simulink model "practica2"  (R2014a)
settings: Solver=ode45  StartTime=0.0  StopTime=10.0  RelTol=1e-3
undefined symbols (not defined in the file): get
libraries: dsparch4 x2, dspsrcs4 x2, dspspect3 x1, dspsnks4 x1
settings Model: Creator=MANU  LastModifiedBy=Isabela

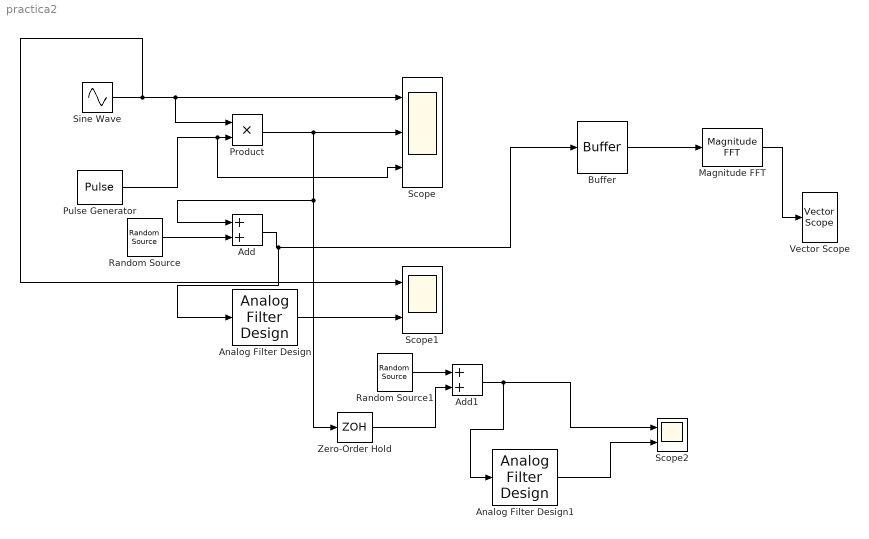
== system practica2 ==
  Add : Sum
  Add1 : Sum
  Analog Filter Design : dsparch4/Analog Filter Design  method=Butterworth  filttype=Lowpass  N=80  Wlo=30  Whi=80  Rp=2  Rs=40
  Analog Filter Design1 : dsparch4/Analog Filter Design  method=Butterworth  filttype=Lowpass  N=30  Wlo=200  Whi=80  Rp=2  Rs=40
  Buffer : Buffer  TreatMby1Signals=One channel
  Magnitude FFT : dspspect3/Magnitude FFT  mag_or_magsq=Magnitude squared  FFTImplementation=Auto  fftLenInherit=off  fftsize=256  WrapInput=on
  Product : Product  RndMeth=Zero
  Pulse Generator : DiscretePulseGenerator  Amplitude=2  Period=3  SampleTime=0.01
  Random Source : dspsrcs4/Random Source  SrcType=Gaussian  NormMethod=Sum of uniform values  CltLength=4  MinVal=0  MaxVal=2  MeanVal=0  VarVal=0.5  RepMode=Not repeatable  rawSeed=1  IsInherit=off  SampMode=Discrete  SampTime=1  SampFrame=1  DataType=Double  OutComplex=Real
  Random Source1 : dspsrcs4/Random Source  SrcType=Gaussian  NormMethod=Sum of uniform values  CltLength=4  MinVal=0  MaxVal=2  MeanVal=0  VarVal=0.5  RepMode=Not repeatable  rawSeed=1  IsInherit=off  SampMode=Discrete  SampTime=1  SampFrame=1  DataType=Double  OutComplex=Real
  Scope : Scope  NumInputPorts=3
      settings: YMin=-5~-5~-5  YMax=5~5~5
  Scope1 : Scope  NumInputPorts=2
      settings: YMin=-5~-5  YMax=5~5
  Scope2 : Scope  NumInputPorts=2
      settings: YMin=-5~-5  YMax=5~5  SaveName=ScopeData2
  Sine Wave : Sin  SineType=Sample based  Amplitude=10  Frequency=5  Samples=60  SampleTime=0.01
  Vector Scope : dspsnks4/Vector Scope  ScopeProperties=on  Domain=Time  HorizSpan=1  DisplayProperties=off  AxisGrid=on  Memory=off  FrameNumber=on  AxisLegend=off  AxisZoom=off  OpenScopeAtSimStart=on  OpenScopeImmediately=off  FigPos=get(0,'defaultfigureposition')  AxisProperties=off  XUnits=Hertz  XRange=[0...Fs/2]  InheritXIncr=on  XIncr=1  XLabel=Time  XLimit=Auto  XMin=0  XMax=1  XStart=0  YUnits=dB  YLabel=Amplitude  LineProperties=off  XAxisParamsVer=6.9
      settings: YMin=-10  YMax=10
  Zero-Order Hold : ZeroOrderHold  SampleTime=0.25
  wires:
  Sine Wave/1 -> Scope1/1, Product/1, Scope/1
  Product/1 -> Zero-Order Hold/1, Add/1, Scope/2
  Analog Filter Design/1 -> Scope1/2
  Analog Filter Design1/1 -> Scope2/2
  Pulse Generator/1 -> Scope/3, Product/2
  Add/1 -> Analog Filter Design/1, Buffer/1
  Random Source/1 -> Add/2
  Magnitude FFT/1 -> Vector Scope/1
  Buffer/1 -> Magnitude FFT/1
  Random Source1/1 -> Add1/1
  Zero-Order Hold/1 -> Add1/2
  Add1/1 -> Analog Filter Design1/1, Scope2/1
